simulink model "piezoelecmarche5"  (R2013a)
settings: Solver=ode45  StartTime=0.0  StopTime=10  RelTol=1e-3
undefined symbols (not defined in the file): sigbuilder_block
libraries: fl_lib x9, nesl_utility x3, elec_lib x1
settings Model: Creator=pc  LastModifiedBy=pc

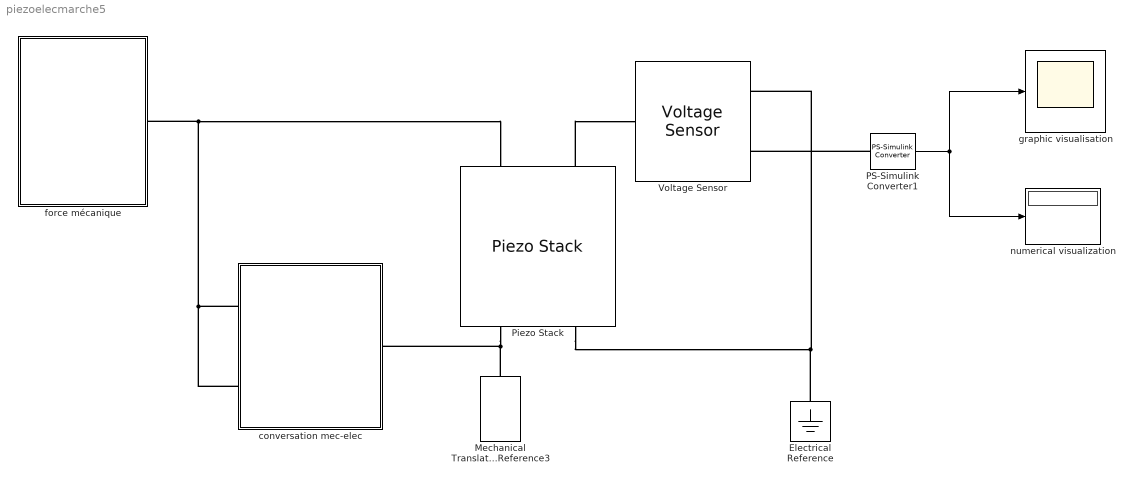
== system piezoelecmarche5 ==
  Electrical Reference : fl_lib/Electrical/Electrical Elements/Electrical Reference  i_Log=off  LocalVarNames=|i  LocalVarDescs=|i  LocalVarLogging=0
  Mechanical Translational Reference3 : fl_lib/Mechanical/Translational Elements/Mechanical Translational Reference  f_Log=off  LocalVarNames=|f  LocalVarDescs=|f  LocalVarLogging=0
  PS-Simulink Converter1 : nesl_utility/PS-Simulink Converter  PhysicalDomain=network_engine_domain  SubClassName=ps_output  LeftPortType=input  RightPortType=output  PseudoPeriodic=off  Frequencies=[]  Unit=V  AffineConversion=off
  Piezo Stack : elec_lib/Actuators & Drivers/Translational Actuators/Piezo Stack  param=1  A=50 mm^2  L0=30 mm  dL0=0.038 mm  F0=3.8e+3 N  V0=120 V  C0=20 uF  dt=0.3 mm  NL=50  d=5e-10 m/V  epsilon=2.124e-8 F/m  s=1.9e-11 m^2/N  paramDyn=1  f=Inf kHz  Qm=Inf  lam=0 N/(m/s)  Mass=0 g  X0=0 mm  V_ini=0 V  current_Log=off  voltage_Log=off  power_Log=off  force_Log=off  speed_Log=off  LocalVarNames=|current|voltage|power|force|speed  LocalVarDescs=|Current (A)|Voltage (V)|Power (W)|Force (N)|Translational speed (m/s)  LocalVarLogging=[0 0 0 0 0]
  Voltage Sensor : fl_lib/Electrical/Electrical Sensors/Voltage Sensor  i1_Log=off  v1_Log=off  LocalVarNames=|i1|v1  LocalVarDescs=|i1|v1  LocalVarLogging=[0 0]
  conversation mec-elec : Subsystem
  force mécanique : Subsystem
  graphic visualisation : Scope
      settings: TimeRange=10  YMin=-30000  YMax=30000
  numerical visualization : Display
      settings: Decimation=100
  wires:
  PS-Simulink Converter1/1 -> numerical visualization/1, graphic visualisation/1
  connections:
  Piezo Stack/LConn1 -- Voltage Sensor/LConn1
  Piezo Stack/RConn1 -- Voltage Sensor/RConn2 -- Electrical Reference/LConn1
  PS-Simulink Converter1/LConn1 -- Voltage Sensor/RConn1
  conversation mec-elec/LConn1 -- conversation mec-elec/LConn2 -- force mécanique/RConn1 -- Piezo Stack/LConn2
  Piezo Stack/RConn2 -- Mechanical Translational Reference3/LConn1 -- conversation mec-elec/RConn1

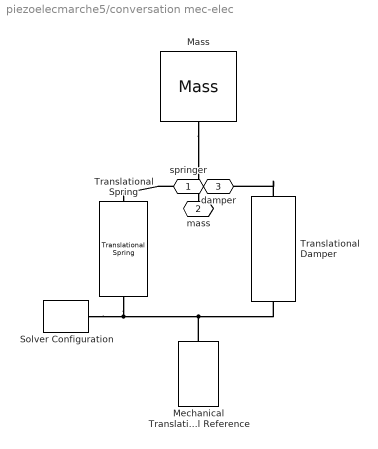
== system piezoelecmarche5/conversation mec-elec ==
  Mass : fl_lib/Mechanical/Translational Elements/Mass  mass=60 kg  initial_velocity=0 m/s  f_Log=off  LocalVarNames=|f  LocalVarDescs=|f  LocalVarLogging=0
  Mechanical Translational Reference : fl_lib/Mechanical/Translational Elements/Mechanical Translational Reference  f_Log=off  LocalVarNames=|f  LocalVarDescs=|f  LocalVarLogging=0
  Solver Configuration : nesl_utility/Solver Configuration  PhysicalDomain=network_engine_domain  SubClassName=solver  LeftPortType=input  RightPortType=generic  Accelerate=off  Tones=[]  Harmonics=[]  SimulateNoise=off  Profile=off  UseLocalSampling=off  EnableSwitchedLinearOptims=on  FrequencyDomain=off  UseCCode=off  UseNewInitialization=off  DoDC=off  ResidualTolerance=1e-09  UseLocalSolver=off  LocalSolverChoice=NE_BACKWARD_EULER_ADVANCER  LocalSolverSampleTime=0.001  DoFixedCost=off  MaxNonlinIter=3  MaxModeIter=2  LinearAlgebra=Sparse  DelaysMemoryBudget=1024
  Translational Damper : fl_lib/Mechanical/Translational Elements/Translational Damper  D=100 N/(m/s)  f_Log=off  v_Log=off  LocalVarNames=|f|v  LocalVarDescs=|f|v  LocalVarLogging=[0 0]
  Translational Spring : fl_lib/Mechanical/Translational Elements/Translational Spring  spr_rate=1000 N/m  init_def=1 cm  f_Log=off  v_Log=off  x_Log=off  LocalVarNames=|f|v|x  LocalVarDescs=|f|v|x  LocalVarLogging=[0 0 0]
  springer : PMIOPort  Port=1  Side=Right
  mass : PMIOPort  Port=2  Side=Left
  damper : PMIOPort  Port=3  Side=Left
  connections:
  Translational Damper/LConn1 -- damper/RConn1
  Translational Spring/RConn1 -- Mechanical Translational Reference/LConn1 -- Translational Damper/RConn1 -- Solver Configuration/RConn1
  Mass/LConn1 -- mass/RConn1
  springer/RConn1 -- Translational Spring/LConn1

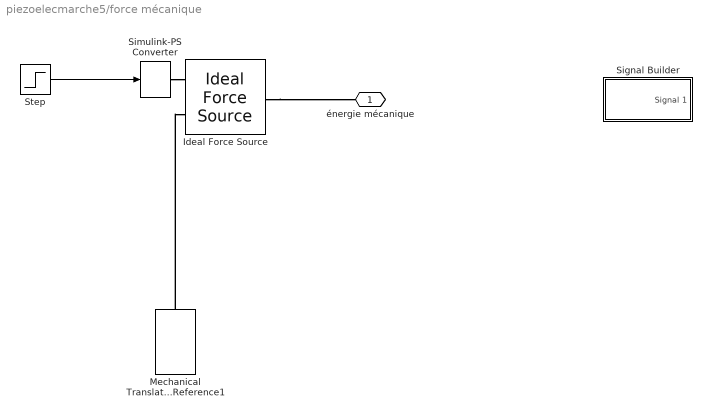
== system piezoelecmarche5/force mécanique ==
  Ideal Force Source : fl_lib/Mechanical/Mechanical Sources/Ideal Force Source  v_Log=off  f_Log=off  LocalVarNames=|v|f  LocalVarDescs=|v|f  LocalVarLogging=[0 0]
  Mechanical Translational Reference1 : fl_lib/Mechanical/Translational Elements/Mechanical Translational Reference  f_Log=off  LocalVarNames=|f  LocalVarDescs=|f  LocalVarLogging=0
  Signal Builder : Subsystem  Tag=STV Subsys  LoadFcn=sigbuilder_block('load');  StartFcn=sigbuilder_block('start');  StopFcn=sigbuilder_block('stop');  ClipboardFcn=sigbuilder_block('clipboard');  mask(Sigbuilder block){}
      mask help: Simulink:masks:SigbuilderBlock_MD
      mask init:
      | if ~strcmp(get_param(bdroot(gcbh),'SimulationStatus'),'stopped') tuvar = sigbuilder_block('maskInit'); end
      settings: CopyFcn=sigbuilder_block('copy');  DeleteFcn=sigbuilder_block('delete');  ModelCloseFcn=sigbuilder_block('modelClose');  PreSaveFcn=sigbuilder_block('preSave');  PauseFcn=sigbuilder_block('pause');  ContinueFcn=sigbuilder_block('continue');  NameChangeFcn=sigbuilder_block('namechange');  OpenFcn=sigbuilder_block('open',[437.25 117.75 550.5 394.5 ]);  CloseFcn=sigbuilder_block('close');
      mask Display: plot(0, 0, 100, 100,[2, 2, 32, 32, 2], [68, 8, 8, 68, 68],[32, 2], [38, 38], [32, 19, 2],[53, 60, 44], [32, 17, 17, 2],[16, 16, 31, 31]);txt = getActiveGroup(gcbh);text(2, 100, txt,'verticalAlignment', 'top');
  Simulink-PS Converter : nesl_utility/Simulink-PS Converter  PhysicalDomain=network_engine_domain  SubClassName=ps_input  LeftPortType=input  RightPortType=output  PseudoPeriodic=off  Frequencies=[]  NoiseDistribution=none  NoiseParameters=[]  Unit=N  AffineConversion=off  InputFiltering=off  SimscapeFilterOrder=1  InputFilterTimeConstant=0.001  UdotUserProvided=1
  Step : Step  Time=0  After=-50  SampleTime=0
  énergie mécanique : PMIOPort  Port=1  Side=Right
  wires:
  Step/1 -> Simulink-PS Converter/1
  connections:
  Simulink-PS Converter/RConn1 -- Ideal Force Source/RConn1
  Mechanical Translational Reference1/LConn1 -- Ideal Force Source/RConn2
  Ideal Force Source/LConn1 -- énergie mécanique/RConn1

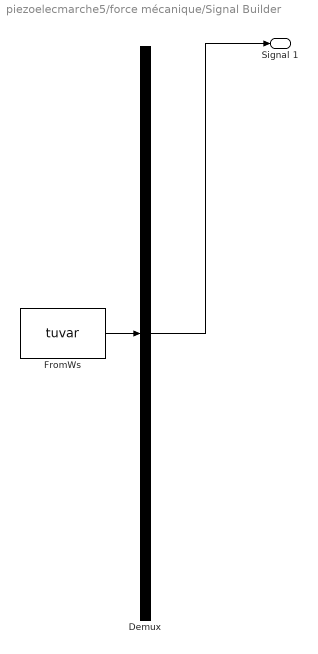
== system piezoelecmarche5/force mécanique/Signal Builder ==
  Demux : Demux  Tag=STV Demux  Outputs=1
  FromWs : FromWorkspace  Tag=STV FromWs  VariableName=tuvar  SampleTime=0
      SigBuilderData=|
      | common.afterFinalStr = 'Extrapolate'
      | common.sampleTime = 0
      | dataSet.timeRange = [0 10]
      | dataSet.name = 'Group 1'
      | sbobj.Groups.Name = 'Group 1'
      | sbobj.Groups.Signals.Name = 'Signal 1'
      | sbobj.Groups.Signals.XData = [0 2.04 2.04 5.98 5.98 10]
      | sbobj.Groups.Signals.YData = [0 0.5 50 50 0 0]
  Signal 1 : Outport  Tag=STV Outport
  wires:
  Demux/1 -> Signal 1/1
  FromWs/1 -> Demux/1
